simulink subsystem "Subsystem_Leds"  (R2023b)
settings: Solver=VariableStepAuto  StartTime=0.0  StopTime=10.0  RelTol=1e-3
libraries: arduinolib x3, simulink x1
settings Model: Creator=Alberto  LastModifiedBy=Alberto

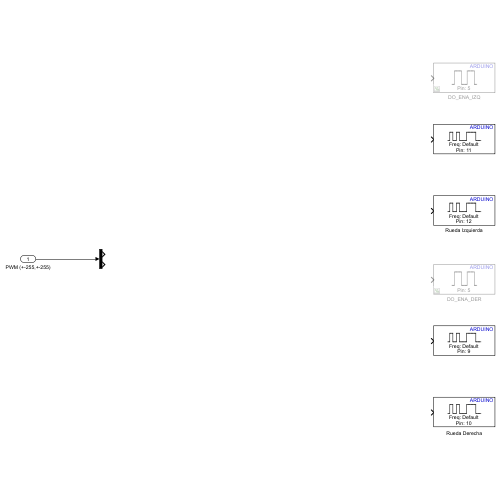
[thumbnail: Simulink's stored preview of the top-level diagram]
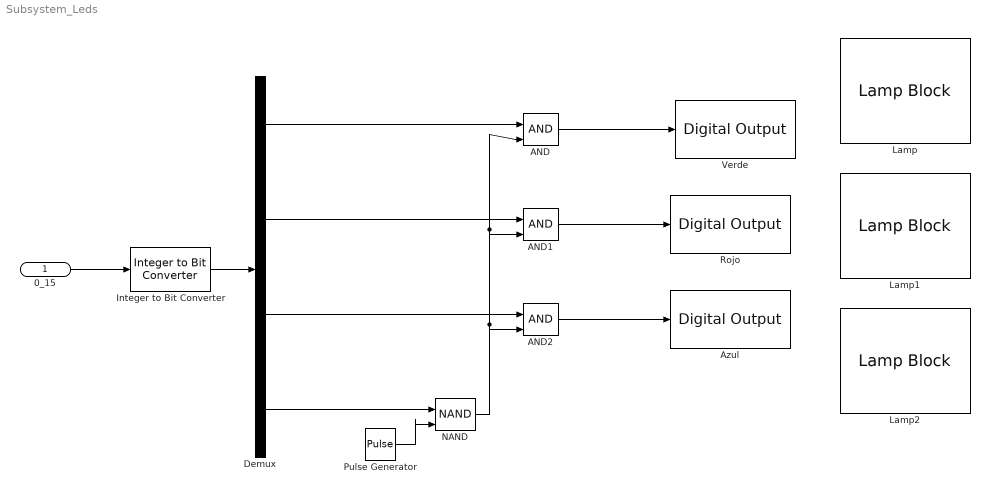
== system Subsystem_Leds ==
  0_15 : Inport
  AND : Logic  IconShape=distinctive  AllPortsSameDT=off  OutDataTypeStr=boolean
  AND1 : Logic  IconShape=distinctive  AllPortsSameDT=off  OutDataTypeStr=boolean
  AND2 : Logic  IconShape=distinctive  AllPortsSameDT=off  OutDataTypeStr=boolean
  Azul : arduinolib/Digital Output  pinNumber=49  Direction=output  blockPlatform=arduino
  Demux : Demux
  Integer to Bit Converter : simulink/Logic and Bit Operations/Integer to Bit Converter  nbits=4  signedInputValues=Unsigned  bitOrder=LSB first  outDtype=boolean
  Lamp : LampBlock  LabelPosition=Hide
  Lamp1 : LampBlock  LabelPosition=Hide
  Lamp2 : LampBlock  LabelPosition=Hide
  NAND : Logic  Operator=NAND  IconShape=distinctive  AllPortsSameDT=off  OutDataTypeStr=boolean
  Pulse Generator : DiscretePulseGenerator  PulseType=Time based  Period=1  PulseWidth=50
  Rojo : arduinolib/Digital Output  pinNumber=51  Direction=output  blockPlatform=arduino
  Verde : arduinolib/Digital Output  pinNumber=53  Direction=output  blockPlatform=arduino
  wires:
  AND/1 -> Verde/1
  AND1/1 -> Rojo/1
  AND2/1 -> Azul/1
  0_15/1 -> Integer to Bit Converter/1
  Integer to Bit Converter/1 -> Demux/1
  Demux/1 -> AND/1
  Demux/2 -> AND1/1
  Demux/3 -> AND2/1
  NAND/1 -> AND2/2, AND1/2, AND/2
  Pulse Generator/1 -> NAND/2
  Demux/4 -> NAND/1
